simulink model "mainor_demo_test"  (R2023a)
settings: Solver=VariableStepAuto  StartTime=0.0  StopTime=50  RelTol=1e-3
settings Model: Creator=Hp  LastModifiedBy=Hp

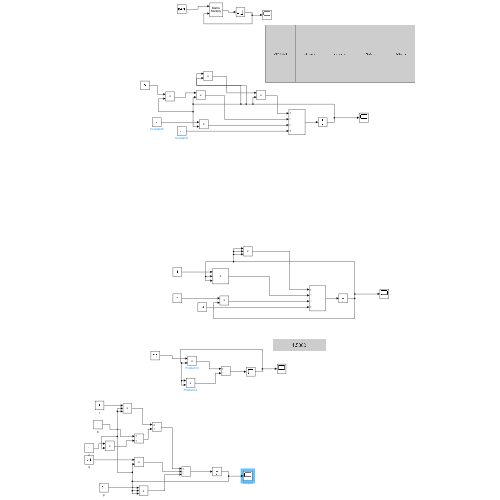
[thumbnail: Simulink's stored preview of the top-level diagram]
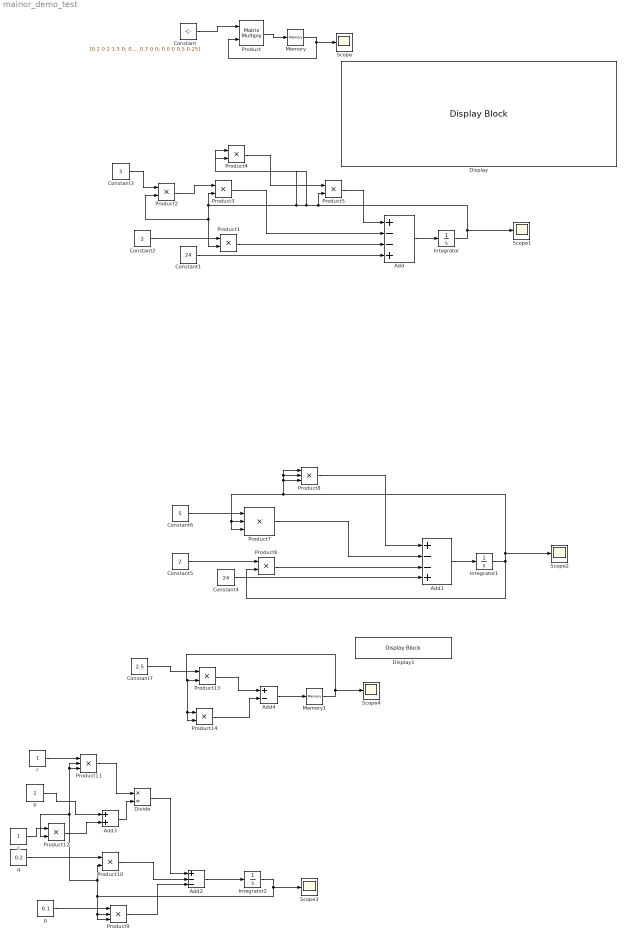
== system mainor_demo_test ==
  Add : Sum  Inputs=+--+
  Add1 : Sum  Inputs=+--+
  Add2 : Sum  Inputs=+--
  Add3 : Sum
  Add4 : Sum  Inputs=+-
  Constant : Constant  Value=[0.2 0 2 1.5 0; 0.6 0 0 0 0; 0 0.9 0 0 0; 0 0 0.7 0 0; 0 0 0 0.5 0.25]
  Constant1 : Constant  Value=24
  Constant2 : Constant  Value=2
  Constant3 : Constant  Value=5
  Constant4 : Constant  Value=24
  Constant5 : Constant  Value=2
  Constant6 : Constant  Value=5
  Constant7 : Constant  Value=2.5
  Display : DisplayBlock  LabelPosition=Hide  Transparency=1
  Display1 : DisplayBlock  LabelPosition=Hide  Transparency=1
  Divide : Product  Inputs=*/
  Integrator : Integrator
  Integrator1 : Integrator
  Integrator2 : Integrator  InitialCondition=6
  Memory : Memory  InitialCondition=[500; 1000; 500; 800; 1200]
  Memory1 : Memory  InitialCondition=1.7
  Product : Product  Multiplication=Matrix(*)
  Product{1..6,10,12..14} (10 alike) : Product
  Product{7..9,11} (4 alike) : Product  Inputs=3
  Scope{,1..4} (5 alike) : Scope
  b : Constant
  c : Constant
  p : Constant  Value=0.1
  q : Constant  Value=0.2
  r : Constant
  wires:
  Constant/1 -> Product/1
  Product/1 -> Memory/1
  Memory/1 -> Scope/1, Product/2
  Add/1 -> Integrator/1
  Constant1/1 -> Add/4
  Constant2/1 -> Product1/1
  Integrator/1 -> Product5/2, Product4/1, Product4/2, Product2/2, Product1/2, Product3/2, Scope1/1
  Product1/1 -> Add/3
  Constant3/1 -> Product2/1
  Product2/1 -> Product3/1
  Product3/1 -> Add/2
  Product4/1 -> Product5/1
  Product5/1 -> Add/1
  Constant5/1 -> Product6/1
  Product6/1 -> Add1/3
  Constant4/1 -> Add1/4
  Add1/1 -> Integrator1/1
  Integrator1/1 -> Product8/1, Product8/2, Product8/3, Product7/3, Product7/2, Scope2/1, Product6/2
  Constant6/1 -> Product7/1
  Product7/1 -> Add1/2
  Product8/1 -> Add1/1
  Add2/1 -> Integrator2/1
  p/1 -> Product9/1
  Integrator2/1 -> Scope3/1, Product12/2, Product11/3, Product11/2, Product10/2, Product9/3, Product9/2
  Product9/1 -> Add2/3
  q/1 -> Product10/1
  Product10/1 -> Add2/2
  r/1 -> Product11/1
  Product11/1 -> Divide/1
  b/1 -> Add3/1
  c/1 -> Product12/1
  Product12/1 -> Add3/2
  Add3/1 -> Divide/2
  Divide/1 -> Add2/1
  Product13/1 -> Add4/1
  Constant7/1 -> Product13/1
  Product14/1 -> Add4/2
  Add4/1 -> Memory1/1
  Memory1/1 -> Scope4/1, Product14/2, Product14/1, Product13/2
